simulink model "KF2"  (R2021a)
settings: Solver=VariableStepAuto  StartTime=0.0  StopTime=40  RelTol=1e-3
values from neighbouring files (symbols this model uses):
  A = sys_d.A    [Script.m]
  B = sys_d.B    [Script.m]
  bias_init = 0    [Script.m]
  C = sys_d.C    [Script.m]
  R = 1000    [Script.m]
  sys_d = c2d(sys,0.02)    [Script.m]
  zsimu = [vztime', zsamp.*cosd(pitch)]    [Script.m]
undefined symbols (not defined in the file or in its folder): Discrete, m, Time
libraries: ctrlSharedLib x1
settings Model: Creator=Simão Amaro  LastModifiedBy=simao

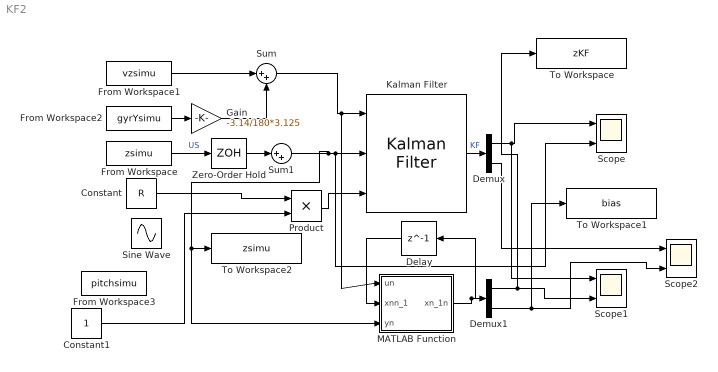
== system KF2 ==
  Constant : Constant  Value=R
  Constant1 : Constant
  Delay : Delay  DelayLength=1  InitialCondition=[zsimu(1,2);bias_init]  SampleTime=0.02
  Demux : Demux  Outputs=2
  Demux1 : Demux  Outputs=2
  From Workspace : FromWorkspace  VariableName=zsimu  SampleTime=0.02
  From Workspace1 : FromWorkspace  VariableName=vzsimu  SampleTime=0.02
  From Workspace2 : FromWorkspace  VariableName=gyrYsimu  SampleTime=0.02
  From Workspace3 : FromWorkspace  VariableName=pitchsimu  SampleTime=0.02
  Gain : Gain  Gain=-3.14/180*3.125
  Kalman Filter : ctrlSharedLib/Kalman Filter  TimeDomain=Discrete-Time  UseCurrentEstimator=on  ModelSource=Individual A, B, C, D matrices  ModelSourceVariable=ss(A,1,1,0,1)  A=sys_d.A  B=sys_d.B  C=sys_d.C  D=sys_d.D  NumberOfStates=1  NumberOfInputs=1  NumberOfOutputs=1  InitialEstimateSource=Dialog  X0=[zsimu(1,2);bias_init]  P0=10  UseK=off  UseGH=off  NumberOfProcessNoiseInputs=1  G=1  TimeInvariantG=on  H=0  TimeInvariantH=on  Q=Q  TimeInvariantQ=on  R=R  TimeInvariantR=off  N=0  TimeInvariantN=on  AddInputPort=on  AddEnablePort=off  OutputEstimatedY=off  OutputP=off  Ts=0.02
  MATLAB Function : MATLAB Function  TreatAsAtomicUnit=on
  Product : Product
  Scope : Scope  NumInputPorts=2
  Scope1 : Scope  NumInputPorts=2
  Scope2 : Scope  NumInputPorts=2
  Sine Wave : Sin  Amplitude=0.2  Frequency=5  SampleTime=0.02
  Sum : Sum  Inputs=|++
  Sum1 : Sum  Inputs=|++
  To Workspace : ToWorkspace  VariableName=zKF  SaveFormat=Timeseries  SampleTime=0.02
  To Workspace1 : ToWorkspace  VariableName=bias  SaveFormat=Timeseries  SampleTime=0.02
  To Workspace2 : ToWorkspace  VariableName=zsimu  SaveFormat=Timeseries  SampleTime=0.02
  Zero-Order Hold : ZeroOrderHold  SampleTime=0.02
  wires:
  From Workspace/1 -> Zero-Order Hold/1  "US"
  Sum/1 -> MATLAB Function/1(un), Kalman Filter/1
  From Workspace2/1 -> Gain/1
  From Workspace1/1 -> Sum/1
  Kalman Filter/1 -> Demux/1  "KF"
  Demux/1 -> Scope1/1, Scope/1
  Demux/2 -> Scope2/1
  MATLAB Function/1(xn_1n) -> Delay/1, Demux1/1
  Delay/1 -> MATLAB Function/2(xnn_1)
  Demux1/1 -> To Workspace/1, Scope1/2
  Demux1/2 -> Scope2/2, To Workspace1/1
  Zero-Order Hold/1 -> Sum1/1
  Sum1/1 -> MATLAB Function/3(yn), To Workspace2/1, Scope/2, Kalman Filter/2
  Constant/1 -> Product/1
  Product/1 -> Kalman Filter/3
  Constant1/1 -> Product/2
  Gain/1 -> Sum/2

== matlab function KF2/MATLAB Function ==
  data: un input; xnn_1 input; yn input; xn_1n output; m parameter; A parameter; B parameter; C parameter
function xn_1n = fcn(un,xnn_1,yn,m, A, B, C)

xnn   = xnn_1 + m*(yn - C*xnn_1);
xn_1n = A*xnn + B*un;
